simulink model "Minimum_snap_trajectory"  (R2021a)
settings: Solver=VariableStepAuto  StartTime=0.0  StopTime=T_s  RelTol=1e-3
values from neighbouring files (symbols this model uses):
  a_x = [0 0 0 0]    [starting_and_end_points.m]
  a_y = [10 40 30 10]    [starting_and_end_points.m]
  a_z = [30 30 30 30]    [starting_and_end_points.m]
  b_x = [0 0 0 0]    [starting_and_end_points.m]
  b_y = [40 30 10 3]    [starting_and_end_points.m]
  b_z = [30 30 30 30]    [starting_and_end_points.m]
  T = 2*max(A)    [starting_and_end_points.m]
libraries: simulink x1
settings Model: Creator=Vogayer  LastModifiedBy=Vogayer

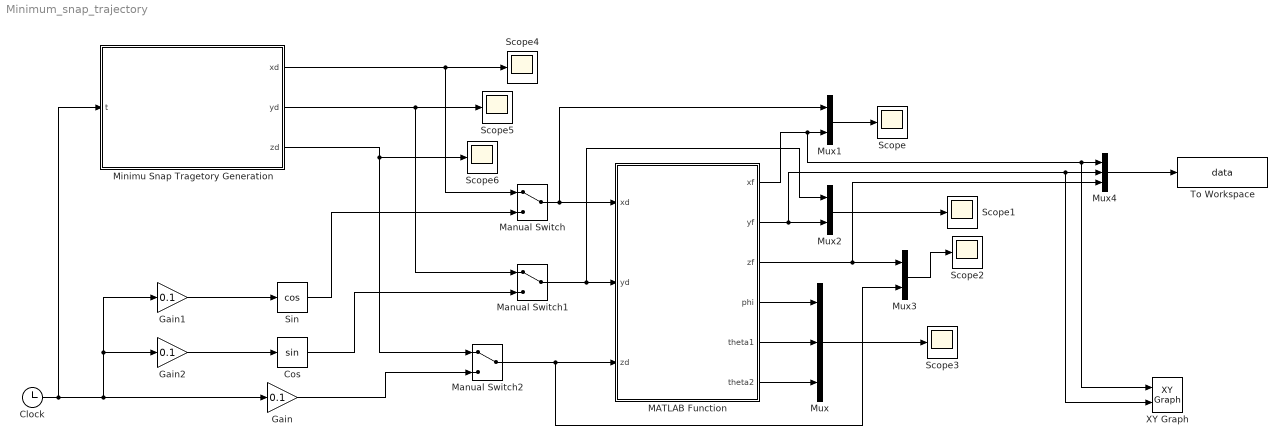
== system Minimum_snap_trajectory ==
  Clock : Clock
  Cos : Trigonometry
  Gain : Gain  Gain=0.1
  Gain1 : Gain  Gain=0.1
  Gain2 : Gain  Gain=0.1
  MATLAB Function : MATLAB Function  TreatAsAtomicUnit=on
  Manual Switch : ManualSwitch
  Manual Switch1 : ManualSwitch
  Manual Switch2 : ManualSwitch
  Minimu Snap Tragetory Generation : Subsystem
  Mux : Mux  Inputs=3
  Mux1 : Mux  Inputs=2
  Mux2 : Mux  Inputs=2
  Mux3 : Mux  Inputs=2
  Mux4 : Mux  Inputs=3
  Scope{,1..6} (7 alike) : Scope
  Sin : Trigonometry  Operator=cos
  To Workspace : ToWorkspace  VariableName=data  SampleTime=-1
  XY Graph : simulink/Sinks/XY Graph  xmin=-1  xmax=1  ymin=-1  ymax=1  st=-1
  wires:
  MATLAB Function/4(phi) -> Mux/1
  MATLAB Function/5(theta1) -> Mux/2
  MATLAB Function/6(theta2) -> Mux/3
  Mux/1 -> Scope3/1
  MATLAB Function/1(xf) -> XY Graph/1, Mux4/1, Mux1/2
  Mux1/1 -> Scope/1
  MATLAB Function/2(yf) -> XY Graph/2, Mux4/2, Mux2/2
  Mux2/1 -> Scope1/1
  Mux3/1 -> Scope2/1
  MATLAB Function/3(zf) -> Mux4/3, Mux3/1
  Clock/1 -> Minimu Snap Tragetory Generation/1(t), Gain/1, Gain1/1, Gain2/1
  Gain2/1 -> Cos/1
  Gain1/1 -> Sin/1
  Cos/1 -> Manual Switch1/2
  Minimu Snap Tragetory Generation/1(xd) -> Manual Switch/1, Scope4/1
  Manual Switch/1 -> MATLAB Function/1(xd), Mux1/1
  Sin/1 -> Manual Switch/2
  Minimu Snap Tragetory Generation/2(yd) -> Scope5/1, Manual Switch1/1
  Manual Switch1/1 -> Mux2/1, MATLAB Function/2(yd)
  Manual Switch2/1 -> Mux3/2, MATLAB Function/3(zd)
  Minimu Snap Tragetory Generation/3(zd) -> Scope6/1, Manual Switch2/1
  Gain/1 -> Manual Switch2/2
  Mux4/1 -> To Workspace/1

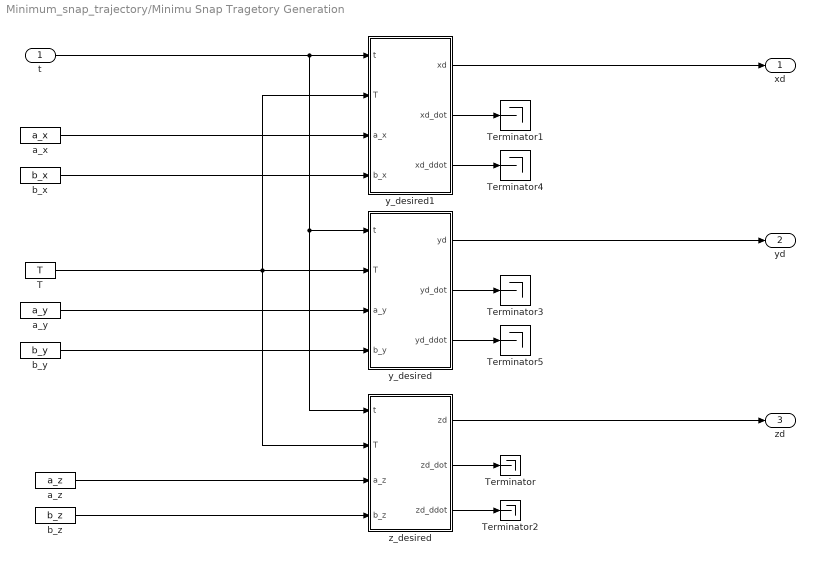
== system Minimum_snap_trajectory/Minimu Snap Tragetory Generation ==
  t : Inport
  " z_desired" : MATLAB Function  TreatAsAtomicUnit=on
  T : Constant  Value=T
  Terminator{,1..5} (6 alike) : Terminator
  a_x : Constant  Value=a_x
  a_y : Constant  Value=a_y
  a_z : Constant  Value=a_z
  b_x : Constant  Value=b_x
  b_y : Constant  Value=b_y
  b_z : Constant  Value=b_z
  y_desired : MATLAB Function  TreatAsAtomicUnit=on
  y_desired1 : MATLAB Function  TreatAsAtomicUnit=on
  xd : Outport
  yd : Outport  Port=2
  zd : Outport  Port=3
  wires:
  " z_desired"/3(zd_ddot) -> Terminator2/1
  " z_desired"/2(zd_dot) -> Terminator/1
  t/1 -> y_desired1/1(t), " z_desired"/1(t), y_desired/1(t)
  y_desired/2(yd_dot) -> Terminator3/1
  a_z/1 -> " z_desired"/3(a_z)
  T/1 -> y_desired1/2(T), " z_desired"/2(T), y_desired/2(T)
  y_desired1/1(xd) -> xd/1
  y_desired/1(yd) -> yd/1
  a_y/1 -> y_desired/3(a_y)
  b_z/1 -> " z_desired"/4(b_z)
  y_desired1/2(xd_dot) -> Terminator1/1
  " z_desired"/1(zd) -> zd/1
  b_y/1 -> y_desired/4(b_y)
  y_desired/3(yd_ddot) -> Terminator5/1
  y_desired1/3(xd_ddot) -> Terminator4/1
  a_x/1 -> y_desired1/3(a_x)
  b_x/1 -> y_desired1/4(b_x)

== matlab function Minimum_snap_trajectory/MATLAB Function ==
  data: xd input; xf output; yd input; zd input; yf output; zf output; phi output; theta1 output; theta2 output
function [xf,yf,zf,phi,theta1,theta2] = fcn(xd,yd,zd)
l1=0.25;l2=4;l3=4;
phi=atan2(yd,xd);
r=sqrt(xd^2 + yd^2);
c2 = (r^2 + (zd-l1)^2 - l2^2 - l3^2)/(2*l2*l3);
s2=sqrt(1 - c2^2);
theta2=atan2(s2,c2);
beta=atan((l3*sin(theta2))/(l2 + l3*cos(theta2)));
gama=atan((zd-l1)/r);
theta1=gama-beta;
rf=l2*cos(theta1) + l3*cos((theta1+theta2));
zf=l1+(l2*sin(theta1) + l3*sin(theta1+theta2));
xf=rf*cos(phi);
yf=rf*sin(phi);

== matlab function Minimum_snap_trajectory/Minimu Snap Tragetory Generation/y_desired1 ==
  data: t input; T input; xd output; xd_dot output; xd_ddot output; a_x input; b_x input
function [xd,xd_dot,xd_ddot] = fcn(t,T,a_x,b_x)
if(t<=T(1,1))
T0=0;Tf=T(1,1);
a=a_x(1,1); b=b_x(1,1);
elseif(t>T(1,1)&& t<=T(2,1)+T(1,1))
T0=T(1,1);Tf=T(2,1)+T(1,1);
a=a_x(2,1); b=b_x(2,1);
elseif (t>T(2,1)+T(1,1)&& t<=T(3,1) + T(2,1)+T(1,1))
T0=T(2,1)+T(1,1);Tf=T(3,1)+ T(2,1)+T(1,1);
a=a_x(3,1); b=b_x(3,1);
else
T0=T(3,1)+ T(2,1)+T(1,1);Tf=T(4,1) + T(3,1)+ T(2,1)+T(1,1);
a=a_x(4,1); b=b_x(4,1);
end
B=[a;b;0;0;0;0;0;0];
A=[T0^6     T0^5     T0^4     T0^3    T0^2  T0^1  1;
   Tf^6     Tf^5     Tf^4     Tf^3    Tf^2  Tf^1  1;
   6*T0^5   5*T0^4   4*T0^3   3*T0^2  2*T0  1     0;
   6*Tf^5   5*Tf^4   4*Tf^3   3*Tf^2  2*Tf  1     0;
   30*T0^4  20*T0^3  12*T0^2  6*T0    2     0     0;
   30*Tf^4  20*Tf^3  12*Tf^2  6*Tf    2     0     0;
   120*T0^3  60*T0^2  24*T0   6       2     0     0;
   120*Tf^3  60*Tf^2  24*Tf   6       2     0     0];
C=A\B;
xd=C(1,1)*t^6 + C(2,1)*t^5 + C(3,1)*t^4 + C(4,1)*t^3 + C(5,1)*t^2 + C(6,1)*t + C(7,1);
xd_dot=6*C(1,1)*t^5 + 5*C(2,1)*t^4  + 4*C(3,1)*t^3 + 3*C(4,1)*t^2 + 2*C(5,1)*t + C(6,1);
xd_ddot=30*C(1,1)*t^4 + 20*C(2,1)*t^3  + 12*C(3,1)*t^2 + 6*C(4,1)*t + 2*C(5,1);

== matlab function Minimum_snap_trajectory/Minimu Snap Tragetory Generation/y_desired ==
  data: t input; T input; yd output; yd_dot output; yd_ddot output; a_y input; b_y input
function [yd,yd_dot,yd_ddot] = fcn(t,T,a_y,b_y)
if(t<=T(1,1))
T0=0;Tf=T(1,1);
a=a_y(1,1); b=b_y(1,1);
elseif(t>T(1,1)&& t<=T(2,1)+T(1,1))
T0=T(1,1);Tf=T(2,1)+T(1,1);
a=a_y(2,1); b=b_y(2,1);
elseif (t>T(2,1)+T(1,1)&& t<=T(3,1) + T(2,1)+T(1,1))
T0=T(2,1)+T(1,1);Tf=T(3,1)+ T(2,1)+T(1,1);
a=a_y(3,1); b=b_y(3,1);
else
T0=T(3,1)+ T(2,1)+T(1,1);Tf=T(4,1) + T(3,1)+ T(2,1)+T(1,1);
a=a_y(4,1); b=b_y(4,1);
end
B=[a;b;0;0;0;0;0;0];
A=[T0^6     T0^5     T0^4     T0^3    T0^2  T0^1  1;
   Tf^6     Tf^5     Tf^4     Tf^3    Tf^2  Tf^1  1;
   6*T0^5   5*T0^4   4*T0^3   3*T0^2  2*T0  1     0;
   6*Tf^5   5*Tf^4   4*Tf^3   3*Tf^2  2*Tf  1     0;
   30*T0^4  20*T0^3  12*T0^2  6*T0    2     0     0;
   30*Tf^4  20*Tf^3  12*Tf^2  6*Tf    2     0     0;
   120*T0^3  60*T0^2  24*T0   6       2     0     0;
   120*Tf^3  60*Tf^2  24*Tf   6       2     0     0];
C=A\B;
yd=C(1,1)*t^6 + C(2,1)*t^5 + C(3,1)*t^4 + C(4,1)*t^3 + C(5,1)*t^2 + C(6,1)*t + C(7,1);
yd_dot=6*C(1,1)*t^5 + 5*C(2,1)*t^4  + 4*C(3,1)*t^3 + 3*C(4,1)*t^2 + 2*C(5,1)*t + C(6,1);
yd_ddot=30*C(1,1)*t^4 + 20*C(2,1)*t^3  + 12*C(3,1)*t^2 + 6*C(4,1)*t + 2*C(5,1);

== matlab function Minimum_snap_trajectory/Minimu Snap Tragetory Generation/ z_desired ==
  data: t input; T input; zd output; zd_dot output; zd_ddot output; a_z input; b_z input
function [zd,zd_dot,zd_ddot] = fcn(t,T,a_z,b_z)
if(t<=T(1,1))
T0=0;Tf=T(1,1);
a=a_z(1,1); b=b_z(1,1);
elseif(t>T(1,1)&& t<=T(2,1)+T(1,1))
T0=T(1,1);Tf=T(2,1)+T(1,1);
a=a_z(2,1); b=b_z(2,1);
elseif (t>T(2,1)+T(1,1)&& t<=T(3,1) + T(2,1)+T(1,1))
T0=T(2,1)+T(1,1);Tf=T(3,1)+ T(2,1)+T(1,1);
a=a_z(3,1); b=b_z(3,1);
else
T0=T(3,1)+ T(2,1)+T(1,1);Tf=T(4,1) + T(3,1)+ T(2,1)+T(1,1);
a=a_z(4,1); b=b_z(4,1);
end
B=[a;b;0;0;0;0;0;0];
A=[T0^6     T0^5     T0^4     T0^3    T0^2  T0^1  1;
   Tf^6     Tf^5     Tf^4     Tf^3    Tf^2  Tf^1  1;
   6*T0^5   5*T0^4   4*T0^3   3*T0^2  2*T0  1     0;
   6*Tf^5   5*Tf^4   4*Tf^3   3*Tf^2  2*Tf  1     0;
   30*T0^4  20*T0^3  12*T0^2  6*T0    2     0     0;
   30*Tf^4  20*Tf^3  12*Tf^2  6*Tf    2     0     0;
   120*T0^3  60*T0^2  24*T0   6       2     0     0;
   120*Tf^3  60*Tf^2  24*Tf   6       2     0     0];
C=A\B;
zd=C(1,1)*t^6 + C(2,1)*t^5 + C(3,1)*t^4 + C(4,1)*t^3 + C(5,1)*t^2 + C(6,1)*t + C(7,1);
zd_dot=6*C(1,1)*t^5 + 5*C(2,1)*t^4  + 4*C(3,1)*t^3 + 3*C(4,1)*t^2 + 2*C(5,1)*t + C(6,1);
zd_ddot=30*C(1,1)*t^4 + 20*C(2,1)*t^3  + 12*C(3,1)*t^2 + 6*C(4,1)*t + 2*C(5,1);
